simulink model "Latest_Greatest_vSandberg"  (R2022b)
settings: Solver=ode4  StartTime=0  StopTime=15  FixedStep=DeltaT  RelTol=1e-6  EnableMultiTasking=on
InitFcn:
  | %run('final_report_initexternal')
  | % Bifocal Relay Mirror Spacecraft (prior to payload installation) Dynamics Simulation          TA Sands
  | clear all;close all;clc;warning off all;
  | 
  | % Simulation run parameters
  | Rate=34.3; Rate=100;  DeltaT=1/Rate;
  | 
  | % Maneuver Parameters
  | roll=0;  pitch=0; yaw=30;   roll=roll*pi/180; pitch=pitch*pi/180; yaw=yaw*pi/180;
  | SlewStart=5; SlewTime=10; SACengage=0;
  | SlewStart=5; SlewTime=5;
  | t0=SlewTime;
  | tf=SlewTime+5;
  | %%
  | 
  | %Constants0
  | Re=6371.2e3;mu=398601.2e9;          %earth radius and universal gravitation constant
  | 
  | % tht=0.5*((sin(pi/SlewTime*(u(4)+2.5)))+1).*[u(1) u(2) u(3)]';
  | % w=(30/77.1239)*0.5*(pi/SlewTime)*((cos(pi/SlewTime*(u(4)+2.5)))+1).*[u(1) u(2) u(3)]'
  | % wdot=-(30/77.1239)*0.5*(pi/SlewTime)^(2)*((sin(pi/SlewTime*(u(4)+2.5)))).*[u(1) u(2) u(3)]'
  | 
  | %compare with differentiating in real time
  | 
  | % A0=[0 0 0];
  | % tht=A0+1/2*(1-cos(pi/SlewTime*(t-SlewStart)))*(A-A0);
  | % w=1/2*(pi/SlewTime)*sin(pi/SlewTime*(t-SlewStart))*(A-A0);
  | % wdot1=1/2*(pi/SlewTime)^2*cos(pi/SlewTime*(t-SlewStart))*(A-A0);
  | 
  | %Spacecraft orbit
  | h=0;                                     %orbit altitude
  | R=Re+h;                             %orbit radius from center of earth
  | we=0.000072921158553;   %earth's angular velocity rad/solar sec(Vallado)
  | wo=sqrt(mu/(Re+h)^3);        %orbit angular velocity
  | incln=36.6001*pi/180;          %Inclination assumed Monterey Latitude
  | epsilon=12*pi/180;  alphao=0;
  | uo=0; nuo=0;                        %Start S/C beneath subsolar point
  | betasun=60; gamma=1.5;
  | a=0.545491852; b=0.314939867;  c=0.704226952;   %Assumed spacecraft rectangular size
  | Area=[b*c a*c a*b];                 %projected area~m^2 in body x,y,z directions
  | density=4.39e-14;
  | kpre=-9.9639/24/3600/180*pi*0;      %nodal precession constant assumed zero here
  | wn=kpre*(Re/(Re+h))^3.5*cos(incln); %nodal precession (zero eccentricity)
  | V=wo*(Re+h);
  | rho=asin(Re/(h+Re));                %earth angular radius
  | Cd=2.5;     psun=4.5E-6;            %Drag coefficient and solar pressure constant~N/m^2
  | Kaero=-0.5*Cd*V^2;   Psolar=2*psun;  %constants for aero and solar torque calculation
  | dL=[0.002 0.002 0.008];             %predicted distance between cp and cg
  | Kme=2.3390e-005;
  | 
  | %Spacecraft Magnetic Properties (assumed)
  | mresid=[0 0 0.01];                  %Spacecraft residual magnetic moment
  | M=mresid;                           %Magnetic unit dipole vector
  | K=7.943e15;
  | 
  | %%
  | % Determining Principal Axes Frame
  | % ACTUAL Spacecraft Inertia conditions
  | Ix=16.67;   Iy=16.67;   Iz=16.67 ;
  | Ixy=0;  Iyz=0;  Ixz=0;
  | ... (+176 lines)
StopFcn:
  | toc
  | %run('final_report_stopexternal')
  | 
  | if flag==0; Hcmg=Hcmg;else;Hcmg=HcmgMP;end;
  | Hxcmg=[];Hycmg=[];Hzcmg=[];CondA=[]; CondA_MP=[];t=[]; SingPt=[];DetA=[];
  | for i=1:max(size(A));  t=[t i*DeltaT];  H=Hcmg(:,:,i); Hx=H(1,:);  Hy=H(2,:);  Hz=H(3,:);
  | detA=det(A(:,1:3,i));Hxcmg=[Hxcmg Hx];  Hycmg=[Hycmg Hy];  Hzcmg=[Hzcmg Hz];
  | CONDA=cond(A(:,:,i));
  | DetA=[DetA detA]; DetA=1./DetA;
  | CondA=[CondA CONDA];end;   %CondA=CondA./max(CondA); DetA=DetA./max(DetA);
  | Hmag=sqrt(Hxcmg.^2+Hycmg.^2+Hzcmg.^2);x=(max(t)-DeltaT);
  | 
  | InvCondA;
  | 
  | if flag==0; MaxInvCond=min(1./CondA(10*Rate+1:end));DELTA=delta;DELTAdot=deltadot;
  | else; MaxInvCond=min(1./CondA_MP(10*Rate+1:end));DELTA=delta_MP;DELTAdot=deltadot_MP;Hcmg=HcmgMP;end;
  | %
  | ERROR=(trajectory*180/pi-Euler);
  | 
  | figure(1); wdotTrajectory=[CMDTrajectory(:,1) CMDTrajectory(:,2) CMDTrajectory(:,3)];  wTrajectory=[CMDTrajectory(:,4) CMDTrajectory(:,5) CMDTrajectory(:,6)]; ThetaTrajectory=180/pi.*[trajectory(:,1) trajectory(:,2) trajectory(:,3)]; set(gca,'fontsize',32, 'fontname','Palatino Linotype');
  | subplot(3,1,1); plot(t,wdotTrajectory, 'linewidth',2); axis tight; grid; ylabel('\omega^d^o^t_C_M_D (deg)','fontsize',32); title('Desired Angle, Rate, Acceleration Trajectories','fontsize',32);   set(gca,'XTick',0:2:15);     set(gca,'XTickLabel',{' ',' ',' ',' ',' ',' ',' ',' ','15'}); set(gca,'fontsize',32, 'fontname','Palatino Linotype');
  | subplot(3,1,2); plot(t,wTrajectory,'linewidth',2); axis tight; grid; ylabel('\omega_C_M_D (deg)','fontsize',32);set(gca,'XTick',0:2:15);     set(gca,'XTickLabel',{' ',' ',' ',' ',' ',' ',' ',' ','15'}); set(gca,'fontsize',32, 'fontname','Palatino Linotype');
  | subplot(3,1,3); plot(t,ThetaTrajectory,'linewidth',2); axis tight; grid; ylabel('\theta_C_M_D (deg)','fontsize',32); xlabel('time (sec)','fontsize',32); set(gca,'fontsize',32, 'fontname','Palatino Linotype');
  | 
  | % figure(2);
  | % subplot(2,1,1);plot(t,Hmag,'LineWidth',3);   ylabel('|H_c_m_g|','Fontsize',16);grid;axis([0,x,0,3]); set(gca,'fontsize',16);set(gca,'XTickLabel',{' ',' ',' ',' ',' ',' ',' ',' ','15'});
  | % subplot(2,1,2);plot(t,InvCondA,'linewidth',3);grid;xlabel('t(sec)','fontsize',14,'fontname','times');ylabel('Cond[A]','fontsize',14,'fontname','times');axis([0,max(t),0,21.82]); set(gca,'fontsize',16);
  | %
  | % DELTA1=DELTA(1,:);DELTA2=DELTA(2,:);DELTA3=DELTA(3,:);DELTA4=DELTA(4,:);
  | % DELTAdot1=DELTAdot(1,:);DELTAdot2=DELTAdot(2,:);DELTAdot3=DELTAdot(3,:);DELTAdot4=DELTAdot(4,:);
  | %
  | % figure(3);subplot(4,1,1);plot(t,DELTA1,'LineWidth',3); title('Gimbal Angles','fontsize',16);ylabel('\theta_1(deg)','Fontsize',14);grid;axis tight; set(gca,'XTickLabel',{' ',' ',' ',' ',' ',' ',' ',' ','15'});set(gca,'fontsize',16);
  | % subplot(4,1,2);plot(t,DELTA2,'LineWidth',3); ylabel('\theta_2(deg)','Fontsize',16);grid;axis tight; set(gca,'XTickLabel',{' ',' ',' ',' ',' ',' ',' ',' ','15'});set(gca,'fontsize',16);
  | % subplot(4,1,3);plot(t,DELTA3,'LineWidth',3); ylabel('\theta_3(deg)','Fontsize',16);grid;axis tight; set(gca,'XTickLabel',{' ',' ',' ',' ',' ',' ',' ',' ','15'});set(gca,'fontsize',16);
  | % subplot(4,1,4);plot(t,InvCondA,'linewidth',3);grid;xlabel('t(sec)','fontsize',14,'fontname','times');ylabel('Cond[A]','fontsize',14,'fontname','times');axis([0,max(t),0,21.82]); set(gca,'fontsize',16);
  | %
  | % figure(4);subplot(4,1,1);plot(t,DELTAdot1,'LineWidth',3);  title('Gimbal Angle RATES','fontsize',16); ylabel('\theta_d_o_t_1(rad/s)','Fontsize',16);grid; axis([0,x,-pi*1.1,pi*1.1]);   set(gca,'XTickLabel',{' ',' ',' ',' ',' ',' ',' ',' ','15'});set(gca,'fontsize',16);
  | % subplot(4,1,2);plot(t,DELTAdot2,'LineWidth',3);   ylabel('\theta_d_o_t_2(rad/s)','Fontsize',16);grid;axis([0,x,-pi*1.1,pi*1.1]);   set(gca,'XTickLabel',{' ',' ',' ',' ',' ',' ',' ',' ','15'});   set(gca,'fontsize',16);
  | % subplot(4,1,3);plot(t,DELTAdot3,'LineWidth',3);   ylabel('\theta_d_o_t_3(rad/s)','Fontsize',16);grid;axis([0,x,-pi*1.1,pi*1.1]); set(gca,'XTickLabel',{' ',' ',' ',' ',' ',' ',' ',' ','15'});set(gca,'fontsize',16);
  | % subplot(4,1,4);plot(t,InvCondA,'linewidth',3);grid;xlabel('t(sec)','fontsize',14,'fontname','times');ylabel('Cond[A]','fontsize',14,'fontname','times');axis([0,max(t),0,21.82]); set(gca,'fontsize',16);
  | %
  | % figure(5);
  | % subplot(4,1,1);plot(t,Hxcmg,'linewidth',3);axis([0,x,-3.25,3.25]);grid;ylabel('h_x/|h|','fontsize',16);title('Normalized Momentum','fontsize',16);set(gca,'XTickLabel',{' ',' ',' ',' ',' ',' ',' ',' ','15'});set(gca,'fontsize',16);
  | % subplot(4,1,2);plot(t,Hycmg,'linewidth',3);axis([0,x,-3.25,3.25]);grid;ylabel('h_y/|h|','fontsize',16);set(gca,'XTickLabel',{' ',' ',' ',' ',' ',' ',' ',' ','15'});set(gca,'fontsize',16);
  | % subplot(4,1,3);plot(t,Hzcmg,'linewidth',3);axis([0,x,-3.25,3.25]);grid;ylabel('h_z/|h|','fontsize',16);  set(gca,'XTickLabel',{' ',' ',' ',' ',' ',' ',' ',' ','15'});set(gca,'fontsize',16);
  | % subplot(4,1,4);plot(t,InvCondA,'linewidth',3);grid;xlabel('t(sec)','fontsize',14,'fontname','times');ylabel('Cond[A]','fontsize',14,'fontname','times');axis([0,max(t),0,21.82]); set(gca,'fontsize',16);
  | %
  | figure(6); EulerX=Euler(:,1);EulerY=Euler(:,2);EulerZ=Euler(:,3);
  | subplot(4,1,1);plot(t,EulerX,'linewidth',3); axis([0,x,min(EulerX),max(EulerX)]);grid;ylabel('\phi(deg)','fontsize',32);title('True Euler Angles','fontsize',14);  set(gca,'XTickLabel',{' ',' ',' ',' ',' ',' ',' ',' ','15'});  set(gca,'fontsize',32, 'fontname','Palatino Linotype');
  | subplot(4,1,2);plot(t,EulerY,'linewidth',3);  axis([0,x,min(EulerY),max(EulerY)]); grid;ylabel('\theta(deg)','fontsize',32);  set(gca,'XTickLabel',{' ',' ',' ',' ',' ',' ',' ',' ','15'}); set(gca,'fontsize',32, 'fontname','Palatino Linotype');
  | subplot(4,1,3);plot(t,EulerZ,'linewidth',3);axis([0,x,min(EulerZ),max(EulerZ)]);grid;  ylabel('\psi(deg)','fontsize',32);  set(gca,'XTickLabel',{' ',' ',' ',' ',' ',' ',' ',' ','15'});  set(gca,'fontsize',32, 'fontname','Palatino Linotype');
  | subplot(4,1,4);plot(t,InvCondA,'linewidth',3);grid;xlabel('t(sec)','fontsize',32,'fontname','times');ylabel('Cond[A]','fontsize',14,'fontname','times');axis([0,max(t),0,21.82]); set(gca,'fontsize',32, 'fontname','Palatino Linotype');
  | 
  | EX=ERROR(:,1);  EY=ERROR(:,2);     EZ=ERROR(:,3);
  | MeanXerror=mean(EX); Xmean=num2str(MeanXerror); xmean=['\mu_\phi=', Xmean];
  | STDx=std(EX);Xsigma=num2str(STDx);SigmaX=['    \sigma_x=' Xsigma];  xlegend=[xmean, SigmaX];
  | MeanYerror=mean(EY); Ymean=num2str(MeanYerror); ymean=['\mu_\theta=', Ymean];
  | STDy=std(EY); Ysigma=num2str(STDy);SigmaY=['    \sigma_y=' Ysigma]; ylegend=[ymean, SigmaY];
  | MeanZerror=mean(EZ); Zmean=num2str(MeanZerror); zmean=['\mu_\psi=', Zmean];
  | STDz=std(EZ);Zsigma=num2str(STDz);SigmaZ=['    \sigma_z=' Zsigma]; zlegend=[zmean, SigmaZ];
  | ... (+113 lines)
undefined symbols (not defined in the file): magnitude, svd
libraries: vrlib x9, dspinverses x8, aerospace x5, matrix_library x4, simulink_need_slupdate x2, dspadpt3 x2
(part 3 of 4)

== system Latest_Greatest_vSandberg/Subsystem2/Subsystem/TAero & Tsolar ==
  note: Taero
  note: Tsolar
  note: Solar and Aero (Drag) Disturbances
  nu : Inport
  DCM : Inport  Port=2
  -1/2CdV^2 : Gain  Gain=-1/2*Cd*V^2  SaturateOnIntegerOverflow=on  OutDataTypeStr=Inherit: Same as input  ParamDataTypeStr=Inherit: Same as input
  2 3x1 cross product : aerospace/Axes Transformations/3x3 cross product
  2 3x1 cross product1 : aerospace/Axes Transformations/3x3 cross product
  Area : Constant  Value=[b*c,a*c,a*b]
  Atmospheric Density @ 800km : Constant  Value=density
  Atmospheric Force in Body Coords : Product  SaturateOnIntegerOverflow=on  OutDataTypeStr=Inherit: Same as first input
  Atmospheric Pressure in Body Coords : Product  SaturateOnIntegerOverflow=on  OutDataTypeStr=Inherit: Same as first input
  On/off : Gain  SaturateOnIntegerOverflow=on  OutDataTypeStr=Inherit: Same as input  ParamDataTypeStr=Inherit: Same as input
  On/off1 : Gain  SaturateOnIntegerOverflow=on  OutDataTypeStr=Inherit: Same as input  ParamDataTypeStr=Inherit: Same as input
  Product1 : Product  SaturateOnIntegerOverflow=on  OutDataTypeStr=Inherit: Same as first input
  Select ci1 : Subsystem
  Solar Force in body coordinates : Product  SaturateOnIntegerOverflow=on  OutDataTypeStr=Inherit: Same as first input
  Solar Pressure : Gain  Gain=Psolar  SaturateOnIntegerOverflow=on  OutDataTypeStr=Inherit: Same as input  ParamDataTypeStr=Inherit: Same as input
  Sum : Sum  SaturateOnIntegerOverflow=on
  Sun & Eclipse : Subsystem
  distance cp to cg : Constant  Value=-dL
  gamma^cos(nu)cos(B)-1 : Fcn  Expr=gamma^(cos(u[1])*cos(betasun)-1)
  Taero & Tsolar : Outport
  wires:
  gamma^cos(nu)cos(B)-1/1 -> Product1/1
  Atmospheric Density @ 800km/1 -> -1/2CdV^2/1
  -1/2CdV^2/1 -> Product1/2
  Solar Pressure/1 -> Solar Force in body coordinates/1
  Area/1 -> Solar Force in body coordinates/2, Atmospheric Force in Body Coords/1
  Product1/1 -> Atmospheric Pressure in Body Coords/1
  Select ci1/1(U(E)) -> Atmospheric Pressure in Body Coords/2
  Atmospheric Pressure in Body Coords/1 -> Atmospheric Force in Body Coords/2
  Solar Force in body coordinates/1 -> 2 3x1 cross product/1
  distance cp to cg/1 -> 2 3x1 cross product/2, 2 3x1 cross product1/2
  Sum/1 -> Taero & Tsolar/1
  Sun & Eclipse/1(Sb) -> Solar Pressure/1
  Sun & Eclipse/2(nu.) -> gamma^cos(nu)cos(B)-1/1
  DCM/1 -> Select ci1/1(U), Sun & Eclipse/2(DCM)
  On/off/1 -> Sum/2
  2 3x1 cross product1/1 -> On/off/1
  2 3x1 cross product/1 -> On/off1/1
  On/off1/1 -> Sum/1
  nu/1 -> Sun & Eclipse/1(nu)
  Atmospheric Force in Body Coords/1 -> 2 3x1 cross product1/1

== system Latest_Greatest_vSandberg/Subsystem2/Subsystem1/Gravity Gradient1 ==
  note: Cant forget that need to divide out by 3 to get the gravitational force
  note: Gravity Gradient Disturbances
  DCM : Inport
  r_body : Inport  Port=2
  3*mu/(norm(r)^3) : MATLABFcn  MATLABFcn=3*mu/norm(u)^3  OutputDimensions=1
  Body Inertia : Gain  Gain=Imo  Multiplication=Matrix(K*u)  SaturateOnIntegerOverflow=on  OutDataTypeStr=Inherit: Same as input  ParamDataTypeStr=Inherit: Same as input
  Cross Product : matrix_library/Cross Product
  Display : Display
  Gain : Gain  Gain=-m/3
  Product : Product
  Product1 : Product
  Select ci3 : Subsystem
  To Workspace2 : ToWorkspace  VariableName=r2  SampleTime=-1
  Tgg : Outport
  Fgg : Outport  Port=2
  wires:
  Gain/1 -> Display/1, Fgg/1
  DCM/1 -> To Workspace2/1, Select ci3/1(U)
  Select ci3/1(U(E)) -> Cross Product/1, Body Inertia/1
  Body Inertia/1 -> Cross Product/2
  Product/1 -> Tgg/1
  r_body/1 -> Product1/2, 3*mu/(norm(r)^3)/1
  Cross Product/1 -> Product/1
  3*mu/(norm(r)^3)/1 -> Product1/1, Product/2
  Product1/1 -> Gain/1

== system Latest_Greatest_vSandberg/Subsystem2/Subsystem1/Magnetic Torque ==
  note: Magnetic Disturbances
  note: Bzo
  note: Byo
  note: Bxo
  DCM : Inport
  alpha : Inport  Port=2
  inclination : Inport  Port=3
  u : Inport  Port=4
  .K/R^3 : Gain  Gain=K/R^3  SaturateOnIntegerOverflow=on  OutDataTypeStr=Inherit: Same as input  ParamDataTypeStr=Inherit: Same as input
  Cross Product : matrix_library/Cross Product
  Cx (orbit coordinates) : Fcn  Expr="cos(u[2])* ( cos(u[4])*sin(u[3])-sin(u[4])*cos(u[3])*cos(u[1])  ) - sin(u[2])*sin(u[4])*sin(u[1])"
  Cx (body coordinates) : Fcn  Expr=u[1]*u[10]+u[2]*u[11]+u[3]*u[12]
  Cy (orbit coordinates) : Fcn  Expr=-cos(u[4])*cos(u[3])-sin(u[4])*sin(u[3])*cos(u[1])
  Cy (body coordinates) : Fcn  Expr=u[4]*u[10]+u[5]*u[11]+u[6]*u[12]
  Cz (orbit coordinates) : Fcn  Expr="2*sin(u[2])*  (cos(u[4])*sin(u[3])-sin(u[4])*cos(u[3])*cos(u[1]) ) + 2*cos(u[2])*sin(u[4])*sin(u[1])"
  Cz (body coordinates) : Fcn  Expr=u[7]*u[10]+u[8]*u[11]+u[9]*u[12]
  Goto1 : Goto  TagVisibility=global
  K/R^3 : Gain  Gain=K/R^3  SaturateOnIntegerOverflow=on  OutDataTypeStr=Inherit: Same as input  ParamDataTypeStr=Inherit: Same as input
  K/R^3. : Gain  Gain=K/R^3  SaturateOnIntegerOverflow=on  OutDataTypeStr=Inherit: Same as input  ParamDataTypeStr=Inherit: Same as input
  Magnetic B Field : Scope  NumInputPorts=3
  Magnetic B Field in Body Coords : Scope
  Magnetic Residual : Constant  Value=M
  Mux : Mux
  Mux1 : Mux
  Mux2 : Mux  Inputs=3
  epsilon : Constant  Value=epsilon
  Sb : Outport
  wires:
  Mux2/1 -> Goto1/1, Magnetic B Field in Body Coords/1, Cross Product/2
  Magnetic Residual/1 -> Cross Product/1
  Cross Product/1 -> Sb/1
  Cz (body coordinates)/1 -> Mux2/3
  Cx (body coordinates)/1 -> Mux2/1
  Cy (body coordinates)/1 -> Mux2/2
  Mux1/1 -> Cz (body coordinates)/1, Cx (body coordinates)/1, Cy (body coordinates)/1
  .K/R^3/1 -> Magnetic B Field/3, Mux1/4
  K/R^3./1 -> Magnetic B Field/2, Mux1/3
  K/R^3/1 -> Magnetic B Field/1, Mux1/2
  DCM/1 -> Mux1/1
  Cz (orbit coordinates)/1 -> .K/R^3/1
  Cy (orbit coordinates)/1 -> K/R^3./1
  Cx (orbit coordinates)/1 -> K/R^3/1
  epsilon/1 -> Mux/4
  Mux/1 -> Cx (orbit coordinates)/1, Cy (orbit coordinates)/1, Cz (orbit coordinates)/1
  inclination/1 -> Mux/3
  alpha/1 -> Mux/2
  u/1 -> Mux/1

== system Latest_Greatest_vSandberg/Subsystem2/Subsystem1/Orbit parameters ==
  note: Orbit parameters
  note: nu=nuo-alpha
  note: alpha
  Clock : Clock
  Sum2 : Sum  Inputs=-+  InputSameDT=on  SaturateOnIntegerOverflow=on  OutDataTypeStr=Inherit: Same as first input
  Sum3 : Sum  InputSameDT=on  SaturateOnIntegerOverflow=on  OutDataTypeStr=Inherit: Same as first input
  Sum4 : Sum  InputSameDT=on  SaturateOnIntegerOverflow=on  OutDataTypeStr=Inherit: Same as first input
  alphao : Constant  Value=alphao
  inclination : Constant  Value=incln
  nuo : Constant  Value=nuo
  udot*t=t/365/360 : Gain  Gain=1/365.242/360  SaturateOnIntegerOverflow=on  OutDataTypeStr=Inherit: Same as input  ParamDataTypeStr=Inherit: Same as input
  uo : Constant  Value=uo
  wo : Gain  Gain=wo  SaturateOnIntegerOverflow=on  OutDataTypeStr=Inherit: Same as input  ParamDataTypeStr=Inherit: Same as input
  alpha : Outport
  incln : Outport  Port=2
  u : Outport  Port=3
  nu : Outport  Port=4
  wires:
  Sum3/1 -> u/1
  inclination/1 -> incln/1
  Sum2/1 -> nu/1
  Sum4/1 -> alpha/1, Sum2/2
  nuo/1 -> Sum2/1
  uo/1 -> Sum3/2
  udot*t=t/365/360/1 -> Sum3/1
  wo/1 -> Sum4/2
  alphao/1 -> Sum4/1
  Clock/1 -> udot*t=t/365/360/1, wo/1

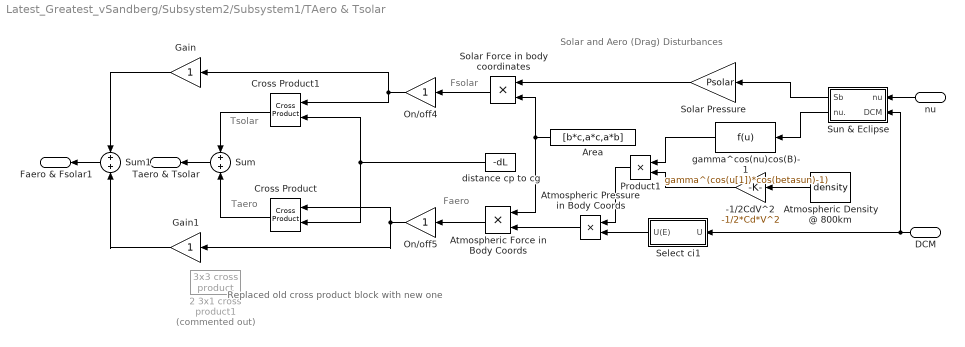
== system Latest_Greatest_vSandberg/Subsystem2/Subsystem1/TAero & Tsolar ==
  note: Fsolar
  note: Faero
  note: Solar and Aero (Drag) Disturbances
  note: Tsolar
  note: Taero
  note: Replaced old cross product block with new one
  nu : Inport
  DCM : Inport  Port=2
  -1/2CdV^2 : Gain  Gain=-1/2*Cd*V^2  SaturateOnIntegerOverflow=on  OutDataTypeStr=Inherit: Same as input  ParamDataTypeStr=Inherit: Same as input
  2 3x1 cross product1 : aerospace/Axes Transformations/3x3 cross product  Commented=on
  Area : Constant  Value=[b*c,a*c,a*b]
  Atmospheric Density @ 800km : Constant  Value=density
  Atmospheric Force in Body Coords : Product  SaturateOnIntegerOverflow=on  OutDataTypeStr=Inherit: Same as first input
  Atmospheric Pressure in Body Coords : Product  SaturateOnIntegerOverflow=on  OutDataTypeStr=Inherit: Same as first input
  Cross Product : vrlib/Utilities/Cross Product
  Cross Product1 : vrlib/Utilities/Cross Product
  Gain : Gain
  Gain1 : Gain
  On/off4 : Gain  SaturateOnIntegerOverflow=on  OutDataTypeStr=Inherit: Same as input  ParamDataTypeStr=Inherit: Same as input
  On/off5 : Gain  SaturateOnIntegerOverflow=on  OutDataTypeStr=Inherit: Same as input  ParamDataTypeStr=Inherit: Same as input
  Product1 : Product  SaturateOnIntegerOverflow=on  OutDataTypeStr=Inherit: Same as first input
  Select ci1 : Subsystem
  Solar Force in body coordinates : Product  SaturateOnIntegerOverflow=on  OutDataTypeStr=Inherit: Same as first input
  Solar Pressure : Gain  Gain=Psolar  SaturateOnIntegerOverflow=on  OutDataTypeStr=Inherit: Same as input  ParamDataTypeStr=Inherit: Same as input
  Sum : Sum  SaturateOnIntegerOverflow=on
  Sum1 : Sum  SaturateOnIntegerOverflow=on
  Sun & Eclipse : Subsystem
  distance cp to cg : Constant  Value=-dL
  gamma^cos(nu)cos(B)-1 : Fcn  Expr=gamma^(cos(u[1])*cos(betasun)-1)
  Taero & Tsolar : Outport
  Faero & Fsolar1 : Outport  Port=2
  wires:
  Gain1/1 -> Sum1/2
  Gain/1 -> Sum1/1
  On/off4/1 -> Gain/1, Cross Product1/1
  On/off5/1 -> Gain1/1, Cross Product/1
  Atmospheric Force in Body Coords/1 -> On/off5/1
  Solar Force in body coordinates/1 -> On/off4/1
  Sum1/1 -> Faero & Fsolar1/1
  nu/1 -> Sun & Eclipse/1(nu)
  Cross Product1/1 -> Sum/1
  Cross Product/1 -> Sum/2
  DCM/1 -> Sun & Eclipse/2(DCM), Select ci1/1(U)
  Sun & Eclipse/2(nu.) -> gamma^cos(nu)cos(B)-1/1
  Sun & Eclipse/1(Sb) -> Solar Pressure/1
  Sum/1 -> Taero & Tsolar/1
  distance cp to cg/1 -> Cross Product/2, Cross Product1/2
  Atmospheric Pressure in Body Coords/1 -> Atmospheric Force in Body Coords/2
  Select ci1/1(U(E)) -> Atmospheric Pressure in Body Coords/2
  Product1/1 -> Atmospheric Pressure in Body Coords/1
  Area/1 -> Solar Force in body coordinates/2, Atmospheric Force in Body Coords/1
  Solar Pressure/1 -> Solar Force in body coordinates/1
  -1/2CdV^2/1 -> Product1/2
  Atmospheric Density @ 800km/1 -> -1/2CdV^2/1
  gamma^cos(nu)cos(B)-1/1 -> Product1/1

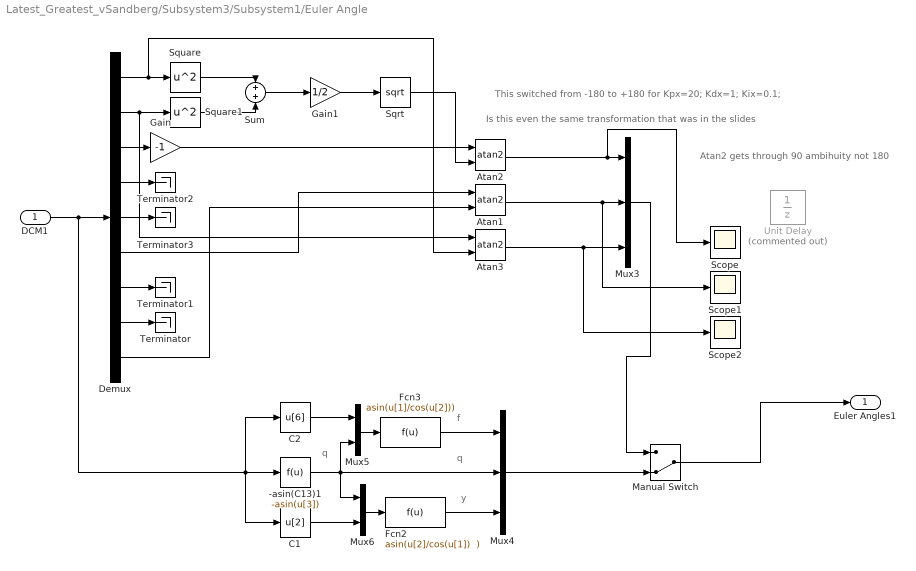
== system Latest_Greatest_vSandberg/Subsystem3/Subsystem1/Euler Angle ==
  note: Atan2 gets through 90 ambihuity not 180
  note: Is this even the same transformation that was in the slides
  note: f
  note: This switched from -180 to +180 for Kpx=20; Kdx=1; Kix=0.1;
  note: q
  note: q
  note: y
  DCM1 : Inport
  -asin(C13)1 : Fcn  Expr=-asin(u[3])
  Atan1 : Trigonometry  Operator=atan2
  Atan2 : Trigonometry  Operator=atan2
  Atan3 : Trigonometry  Operator=atan2
  C1 : Fcn  Expr=u[2]
  C2 : Fcn  Expr=u[6]
  Demux : Demux  Outputs=9
  Fcn2 : Fcn  Expr="asin(u[2]/cos(u[1])  )"
  Fcn3 : Fcn  Expr=asin(u[1]/cos(u[2]))
  Gain : Gain  Gain=-1
  Gain1 : Gain  Gain=1/2
  Manual Switch : ManualSwitch  CurrentSetting=0
  Mux3 : Mux  Inputs=3
  Mux4 : Mux  Inputs=3
  Mux5 : Mux  Inputs=2
  Mux6 : Mux  Inputs=2
  Scope : Scope
  Scope1 : Scope
  Scope2 : Scope
  Sqrt : Sqrt
  Square : Math  Operator=square
  Square1 : Math  Operator=square
  Sum : Sum
  Terminator{,1..3} (4 alike) : Terminator
  Unit Delay : UnitDelay  Commented=on  SampleTime=-1  HasFrameUpgradeWarning=on
  Euler Angles1 : Outport  VectorParamsAs1DForOutWhenUnconnected=off
  wires:
  DCM1/1 -> -asin(C13)1/1, C2/1, C1/1, Demux/1
  Square1/1 -> Sum/2
  -asin(C13)1/1 -> Mux4/2, Mux5/2, Mux6/1
  Gain1/1 -> Sqrt/1
  C2/1 -> Mux5/1
  Fcn3/1 -> Mux4/1
  Demux/3 -> Gain/1
  Mux5/1 -> Fcn3/1
  Mux3/1 -> Manual Switch/1
  Gain/1 -> Atan2/1
  Demux/6 -> Atan1/1
  Mux4/1 -> Manual Switch/2
  Demux/7 -> Terminator1/1
  Sqrt/1 -> Atan2/2
  Demux/9 -> Atan1/2
  C1/1 -> Mux6/2
  Demux/8 -> Terminator/1
  Atan1/1 -> Scope1/1, Mux3/2
  Demux/1 -> Atan3/2, Square/1
  Demux/2 -> Atan3/1, Square1/1
  Square/1 -> Sum/1
  Sum/1 -> Gain1/1
  Fcn2/1 -> Mux4/3
  Demux/5 -> Terminator3/1
  Manual Switch/1 -> Euler Angles1/1
  Demux/4 -> Terminator2/1
  Atan3/1 -> Scope2/1, Mux3/3
  Mux6/1 -> Fcn2/1
  Atan2/1 -> Scope/1, Mux3/1

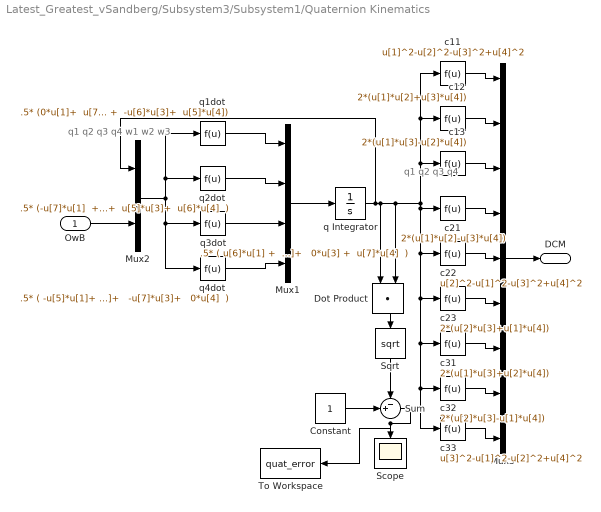
== system Latest_Greatest_vSandberg/Subsystem3/Subsystem1/Quaternion Kinematics ==
  note: q1
      | q2
      | q3
      | q4
      | w1
      | w2
      | w3
  note: q1
      | q2
      | q3
      | q4
  OwB : Inport
  Constant : Constant
  Dot Product : DotProduct  OutDataTypeStr=Inherit: Inherit via internal rule
  Mux1 : Mux
  Mux2 : Mux  Inputs=2
  Mux3 : Mux  Inputs=9
  Scope : Scope
  Sqrt : Sqrt
  Sum : Sum  Inputs=-+|
  To Workspace : ToWorkspace  VariableName=quat_error  SampleTime=-1
  c11 : Fcn  Expr=u[1]^2-u[2]^2-u[3]^2+u[4]^2
  c12 : Fcn  Expr=2*(u[1]*u[2]+u[3]*u[4])
  c13 : Fcn  Expr=2*(u[1]*u[3]-u[2]*u[4])
  c21 : Fcn  Expr=2*(u[1]*u[2]-u[3]*u[4])
  c22 : Fcn  Expr=u[2]^2-u[1]^2-u[3]^2+u[4]^2
  c23 : Fcn  Expr=2*(u[2]*u[3]+u[1]*u[4])
  c31 : Fcn  Expr=2*(u[1]*u[3]+u[2]*u[4])
  c32 : Fcn  Expr=2*(u[2]*u[3]-u[1]*u[4])
  c33 : Fcn  Expr=u[3]^2-u[1]^2-u[2]^2+u[4]^2
  q Integrator : Integrator  InitialCondition=qo
  q1dot : Fcn  Expr=".5* (0*u[1]+  u[7]*u[2] +  -u[6]*u[3]+  u[5]*u[4])"
  q2dot : Fcn  Expr=".5* (-u[7]*u[1]  +  0*u[2]+  u[5]*u[3]+  u[6]*u[4]  )"
  q3dot : Fcn  Expr=".5* ( u[6]*u[1] +  -u[5]*u[2]+   0*u[3] +  u[7]*u[4]  )"
  q4dot : Fcn  Expr=".5* ( -u[5]*u[1]+   -u[6]*u[2]+   -u[7]*u[3]+   0*u[4]  )"
  DCM : Outport  VectorParamsAs1DForOutWhenUnconnected=off
  wires:
  OwB/1 -> Mux2/2
  q1dot/1 -> Mux1/1
  q2dot/1 -> Mux1/2
  q3dot/1 -> Mux1/3
  q4dot/1 -> Mux1/4
  Mux1/1 -> q Integrator/1
  q Integrator/1 -> Dot Product/1, Dot Product/2, c12/1, c11/1, c13/1, c21/1, c22/1, c23/1, c31/1, c33/1, c32/1, Mux2/1
  c11/1 -> Mux3/1
  c12/1 -> Mux3/2
  c13/1 -> Mux3/3
  c22/1 -> Mux3/5
  c21/1 -> Mux3/4
  c23/1 -> Mux3/6
  c31/1 -> Mux3/7
  c32/1 -> Mux3/8
  c33/1 -> Mux3/9
  Mux3/1 -> DCM/1
  Mux2/1 -> q2dot/1, q1dot/1, q3dot/1, q4dot/1
  Dot Product/1 -> Sqrt/1
  Sqrt/1 -> Sum/1
  Sum/1 -> To Workspace/1, Scope/1
  Constant/1 -> Sum/2

== system Latest_Greatest_vSandberg/Subsystem3/Subsystem1/Select ci2 ==
  U : Inport
  C12 : Fcn  Expr=u[2]
  C22 : Fcn  Expr=u[5]
  C32 : Fcn  Expr=u[8]
  Mux2 : Mux  Inputs=3
  U(E) : Outport  VectorParamsAs1DForOutWhenUnconnected=off
  wires:
  C12/1 -> Mux2/1
  C22/1 -> Mux2/2
  C32/1 -> Mux2/3
  U/1 -> C32/1, C22/1, C12/1
  Mux2/1 -> U(E)/1

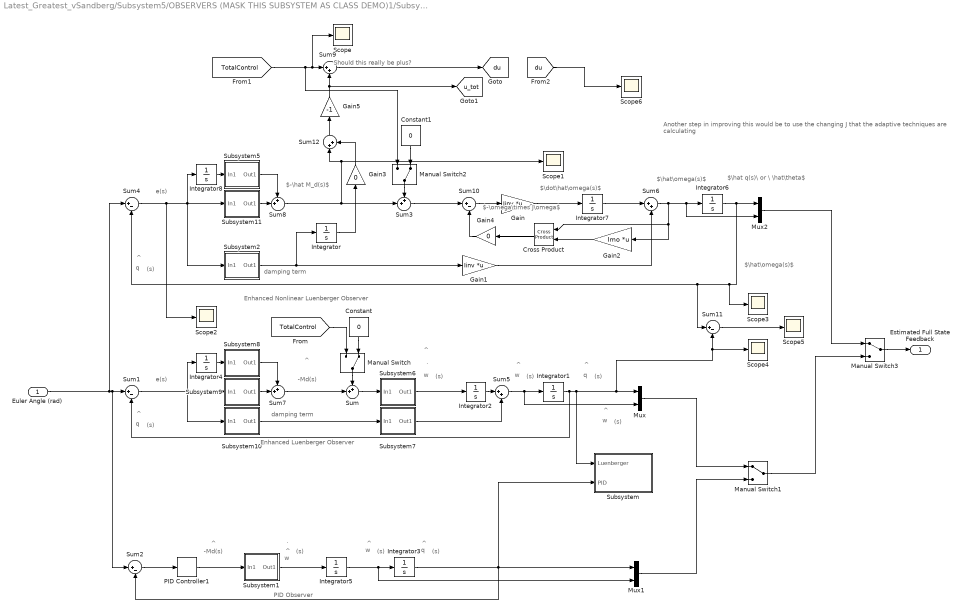
== system Latest_Greatest_vSandberg/Subsystem5/OBSERVERS (MASK THIS SUBSYSTEM AS CLASS DEMO)1/Subsystem ==
  note: Another step in improving this would be to use the changing J that the adaptive techniques are calculating
  note: Should this really be plus?
  note: PID Observer
  note: -Md(s)
  note: ^
  note: ^
  note: (s)
  note: w
  note: (s)
  note: .
  note: ^
  note: w
  note: e(s)
  note: q
  note: ^
  note: (s)
  note: ^
  note: (s)
  note: w
  note: damping term
  note: Enhanced Luenberger Observer
  note: ^
  note: (s)
  note: w
  note: (s)
  note: .
  note: ^
  note: w
  note: (s)
  note: ^
  note: q
  note: ^
  note: -Md(s)
  note: (s)
  note: ^
  note: q
  note: Enhanced Nonlinear Luenberger Observer
  note: $\hat q(s)\ or \ \hat\theta$
  note: q
  note: e(s)
  note: $-\hat M_d(s)$
  note: $\dot\hat\omega(s)$
  note: $\hat\omega(s)$
  note: damping term
  note: (s)
  note: ^
  note: $\hat\omega(s)$
  note: $-\omega\times J\omega$
  Euler Angle (rad) : Inport
  Constant : Constant  Value=0
  Constant1 : Constant  Value=0
  Cross Product : vrlib/Utilities/Cross Product
  Gain : Gain  Gain=Iinv  Multiplication=Matrix(K*u)
  Gain1 : Gain  Gain=Iinv  Multiplication=Matrix(K*u)
  Gain2 : Gain  Gain=Imo  Multiplication=Matrix(K*u)
  Gain3 : Gain  Gain=0
  Gain4 : Gain  Gain=0
  Gain5 : Gain  Gain=-1
  Integrator{,1..8} (9 alike) : Integrator
  Manual Switch : ManualSwitch  CurrentSetting=0
  Manual Switch1 : ManualSwitch
  Manual Switch2 : ManualSwitch  CurrentSetting=0
  Manual Switch3 : ManualSwitch
  Mux : Mux  Inputs=2
  Mux1 : Mux  Inputs=2
  Mux2 : Mux  Inputs=2
  PID Controller1 : simulink_need_slupdate/PID Controller  P=Kpo  I=Kio  D=Kdo
  Scope{,1..6} (7 alike) : Scope
  Subsystem : Subsystem
      mask Display: disp('Scopes')
  Subsystem1 : Subsystem
      mask Display: disp('1/J^p')
  Subsystem10 : Subsystem
      mask Display: disp('Kdo')
  Subsystem11 : Subsystem
      mask Display: disp('Kpo')
  Subsystem2 : Subsystem
      mask Display: disp('Kdo')
  Subsystem5 : Subsystem
      mask Display: disp('Kio')
  Subsystem6 : Subsystem
      mask Display: disp('1/J^p')
  Subsystem7 : Subsystem
      mask Display: disp('1/J^p')
  Subsystem8 : Subsystem
      mask Display: disp('Kio')
  Subsystem9 : Subsystem
      mask Display: disp('Kpo')
  Sum{,3,7..8} (4 alike) : Sum  Inputs=++|
  Sum{1..2,4,10..11} (5 alike) : Sum  Inputs=|+-
  Sum{5..6,9,12} (4 alike) : Sum  Inputs=|++
  Estimated Full State Feedback : Outport  VectorParamsAs1DForOutWhenUnconnected=off
  tag scope: du=global, u_tot=global
  wires:
  Mux1/1 -> Manual Switch1/2
  Mux/1 -> Manual Switch1/1
  PID Controller1/1 -> Subsystem1/1(In1)
  Integrator3/1 -> Mux1/1, Subsystem/2(PID), Sum2/2
  Integrator5/1 -> Mux1/2, Integrator3/1
  Subsystem1/1(Out1) -> Integrator5/1
  Manual Switch/1 -> Sum/1
  Constant/1 -> Manual Switch/2
  [TotalControl] -> Manual Switch/1
  Sum1/1 -> Subsystem10/1(In1), Subsystem9/1(In1), Integrator4/1
  Sum/1 -> Subsystem6/1(In1)
  Sum7/1 -> Sum/2
  Integrator1/1 -> Subsystem/1(Luenberger), Scope4/1, Sum11/2, Mux/1, Sum1/2
  Sum5/1 -> Mux/2, Integrator1/1
  Integrator4/1 -> Subsystem8/1(In1)
  Subsystem10/1(Out1) -> Subsystem7/1(In1)
  Subsystem9/1(Out1) -> Sum7/2
  Subsystem8/1(Out1) -> Sum7/1
  Subsystem7/1(Out1) -> Sum5/2
  Integrator2/1 -> Sum5/1
  Subsystem6/1(Out1) -> Integrator2/1
  Sum2/1 -> PID Controller1/1
  Manual Switch3/1 -> Estimated Full State Feedback/1
  Mux2/1 -> Manual Switch3/1
  Integrator8/1 -> Subsystem5/1(In1)
  [TotalControl] -> Manual Switch2/1, Scope/1, Sum9/1
  Sum8/1 -> Sum12/1, Scope1/1, Sum3/2
  Constant1/1 -> Manual Switch2/2
  Gain1/1 -> Sum6/2
  Subsystem11/1(Out1) -> Sum8/2
  Integrator6/1 -> Mux2/1, Scope3/1, Sum11/1, Sum4/2
  Subsystem2/1(Out1) -> Integrator/1, Gain1/1
  Sum6/1 -> Gain2/1, Cross Product/1, Mux2/2, Integrator6/1
  Euler Angle (rad)/1 -> Sum1/1, Sum2/1, Sum4/1
  Sum4/1 -> Scope2/1, Subsystem2/1(In1), Subsystem11/1(In1), Integrator8/1
  Integrator7/1 -> Sum6/1
  Subsystem5/1(Out1) -> Sum8/1
  Gain/1 -> Integrator7/1
  Manual Switch2/1 -> Sum3/1
  Gain2/1 -> Cross Product/2
  Cross Product/1 -> Gain4/1
  Sum10/1 -> Gain/1
  Sum3/1 -> Sum10/1
  Sum11/1 -> Scope5/1
  [du] -> Scope6/1
  Integrator/1 -> Gain3/1
  Sum9/1 -> [du]
  Gain3/1 -> Sum12/2
  Gain4/1 -> Sum10/2
  Manual Switch1/1 -> Manual Switch3/2
  Sum12/1 -> Gain5/1
  Gain5/1 -> [u_tot], Sum9/2

== system Latest_Greatest_vSandberg/CMGs/Subsystem3/Subsystem1/Subsystem25 ==
  In1 : Inport
  Clock : Clock
  Ki : Gain  Gain=-Ki
  To Workspace : ToWorkspace  VariableName=t  SampleTime=-1
  Out1 : Outport  VectorParamsAs1DForOutWhenUnconnected=off
  wires:
  Clock/1 -> To Workspace/1
  In1/1 -> Ki/1
  Ki/1 -> Out1/1

== system Latest_Greatest_vSandberg/CMGs/Subsystem3/Subsystem1/Subsystem26 ==
  In1 : Inport
  Gain : Gain  Gain=-Kp
  Out1 : Outport  VectorParamsAs1DForOutWhenUnconnected=off
  wires:
  Gain/1 -> Out1/1
  In1/1 -> Gain/1

== system Latest_Greatest_vSandberg/CMGs/Subsystem3/Subsystem1/Subsystem27 ==
  In1 : Inport
  Gain : Gain  Gain=-Kd
  Out1 : Outport  VectorParamsAs1DForOutWhenUnconnected=off
  wires:
  In1/1 -> Gain/1
  Gain/1 -> Out1/1

== system Latest_Greatest_vSandberg/CMGs/Subsystem3/Subsystem4/Subsystem ==
  note: I*wdot+wxI*w
  In1 : Inport
  In2 : Inport  Port=2
  Cross Product : vrlib/Utilities/Cross Product
  Gain : Gain  Gain=Imo  Multiplication=Matrix(K*u)
  Gain1 : Gain  Gain=Imo  Multiplication=Matrix(K*u)
  Sum : Sum  Inputs=|++
  Out1 : Outport
  wires:
  In1/1 -> Gain/1
  Gain1/1 -> Cross Product/2
  Gain/1 -> Sum/1
  Sum/1 -> Out1/1
  In2/1 -> Gain1/1, Cross Product/1
  Cross Product/1 -> Sum/2

== system Latest_Greatest_vSandberg/CMGs/Subsystem3/Subsystem4/Subsystem1 ==
  note: REMAKE THIS< WITH AND WITHOUT REFERENCE
  note: xdotr
  note: xdDot
  note: F
  note: -G
  note: F
  note: s
  note: =
  note: .
  note: ^
  note: q
  omegadot_traj : Inport
  w : Inport  Port=2
  LAMBDA*xtilda : Inport  Port=3
  -G : Gain  Gain=-ETA  SaturateOnIntegerOverflow=on  OutDataTypeStr=Inherit: Same as input  ParamDataTypeStr=Inherit: Same as input
  Derivative2 : Derivative
  F : MATLABFcn  MATLABFcn="[u(1) u(2) u(3) 0 0 0 0 -u(6) u(5);  0 u(1) 0 u(2) u(3) 0 u(6) 0 u(4);  0 0 u(1) 0 u(2) u(3) -u(5) u(4) 0  ]"  OutputDimensions=[27]
  Integrator11 : Integrator  InitialCondition=THETAo
  Manual Switch3 : ManualSwitch
  Math Function : Math  Operator=transpose  SignedPower=on
  Mux : Mux  Inputs=2
  Reshape : Reshape  OutputDimensionality=Customize  OutputDimensions=[3,9]
  Reshape1 : Reshape  OutputDimensions=[1,9]
  Scope{,1..3} (4 alike) : Scope
  Sum2 : Sum  Inputs=|-+  SaturateOnIntegerOverflow=on
  To Workspace : ToWorkspace  VariableName=THETAhat  SampleTime=-1
  To Workspace1 : ToWorkspace  VariableName=CMDTrajectory  SampleTime=-1
  "[F] {q}" : Product  Multiplication=Matrix(*)
  "[PHI] {s}" : Product  Multiplication=Matrix(*)  SaturateOnIntegerOverflow=on  OutDataTypeStr=Inherit: Same as first input
  l : Gain  Gain=LAMBDA  SaturateOnIntegerOverflow=on  OutDataTypeStr=Inherit: Same as input  ParamDataTypeStr=Inherit: Same as input
  l2 : Gain  Gain=uffGain  SaturateOnIntegerOverflow=on  OutDataTypeStr=Inherit: Same as input  ParamDataTypeStr=Inherit: Same as input
  rad2deg : Gain  Gain=180/pi  SaturateOnIntegerOverflow=on  OutDataTypeStr=Inherit: Same as input  ParamDataTypeStr=Inherit: Same as input
  Out1 : Outport
  wires:
  omegadot_traj/1 -> Manual Switch3/1
  Derivative2/1 -> Manual Switch3/2
  Math Function/1 -> "[PHI] {s}"/1
  l/1 -> Sum2/1
  "[PHI] {s}"/1 -> -G/1
  -G/1 -> Integrator11/1
  Reshape1/1 -> To Workspace/1
  Manual Switch3/1 -> Mux/1, Scope1/1
  Sum2/1 -> Scope3/1, "[PHI] {s}"/2
  F/1 -> Reshape/1
  l2/1 -> Out1/1
  Integrator11/1 -> Scope2/1, "[F] {q}"/2, Reshape1/1
  Reshape/1 -> "[F] {q}"/1, Math Function/1
  w/1 -> Sum2/2, Mux/2, Derivative2/1
  rad2deg/1 -> To Workspace1/1
  Mux/1 -> F/1, rad2deg/1
  "[F] {q}"/1 -> Scope/1, l2/1
  LAMBDA*xtilda/1 -> l/1

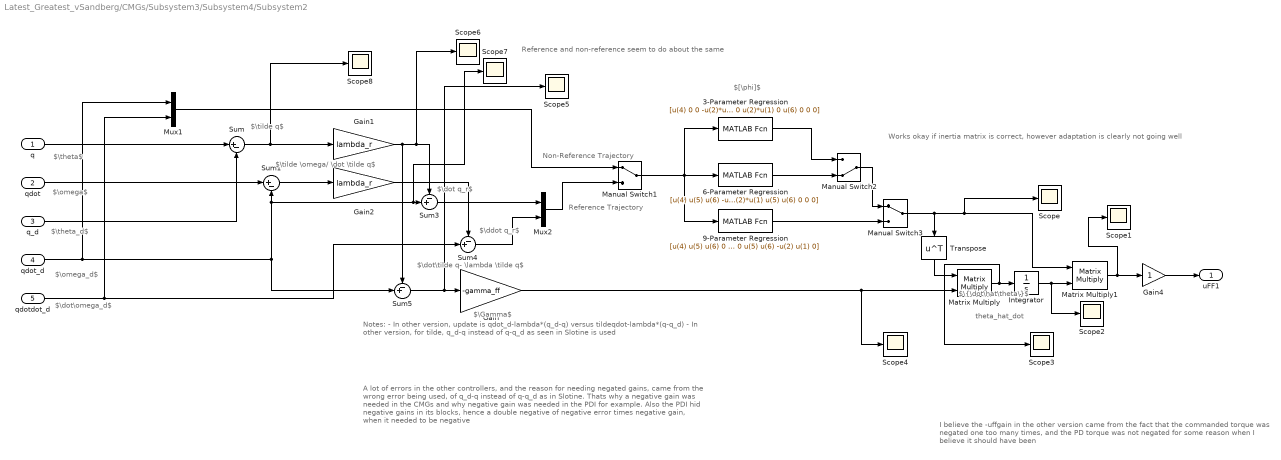
== system Latest_Greatest_vSandberg/CMGs/Subsystem3/Subsystem4/Subsystem2 ==
  note: Reference and non-reference seem to do about the same
  note: A lot of errors in the other controllers, and the reason for needing negated gains, came from the wrong error being used, of q_d-q instead of q-q_d as in Slotine. Thats why a negative gain was needed in the CMGs and why negative gain was needed in the PDI for example. Also the PDI hid negative gains in its blocks, hence a double negative of negative error times negative gain, when it needed to be negative
  note: I believe the -uffgain in the other version came from the fact that the commanded torque was negated one too many times, and the PD torque was not negated for some reason when I believe it should have been
  note: Notes:
      | - In other version, update is qdot_d-lambda*(q_d-q) versus tildeqdot-lambda*(q-q_d)
      | - In other version, for tilde, q_d-q instead of q-q_d as seen in Slotine is used
  note: Works okay if inertia matrix is correct, however adaptation is clearly not going well
  note: theta_hat_dot
  note: $\{\dot\hat\theta\}$
  note: $\Gamma$
  note: $\dot\tilde q- \lambda \tilde q$
  note: $[\phi]$
  note: Non-Reference Trajectory
  note: Reference Trajectory
  note: $\dot q_r$
  note: $\ddot q_r$
  note: $\tilde \omega/ \dot \tilde q$
  note: $\theta$
  note: $\omega$
  note: $\theta_d$
  note: $\omega_d$
  note: $\dot\omega_d$
  note: $\tilde q$
  q : Inport
  qdot : Inport  Port=2
  q_d : Inport  Port=3
  qdot_d : Inport  Port=4
  qdotdot_d : Inport  Port=5
  3-Parameter Regression : MATLABFcn  MATLABFcn=[u(4) 0 0 -u(2)*u(3) 0 u(3)*u(2) 0 0 0;u(1)*u(3) 0 0 u(5) 0 -u(3)*u(1) 0 0 0;-u(1)*u(2) 0 0 u(2)*u(1) 0 u(6) 0 0 0]  Output1D=off
  6-Parameter Regression : MATLABFcn  MATLABFcn=[u(4) u(5) u(6) -u(2)*u(3) 0 u(3)*u(2) 0 0 0;u(1)*u(3) u(4) 0 u(5) u(6) -u(3)*u(1) 0 0 0;-u(1)*u(2) 0 u(4) u(2)*u(1) u(5) u(6) 0 0 0]  Output1D=off
  9-Parameter Regression : MATLABFcn  MATLABFcn=[u(4) u(5) u(6) 0 0 0 0 -u(3) u(2);0 u(4) 0 u(5) u(6) 0 u(3) 0 u(1);0 0 u(4) 0 u(5) u(6) -u(2) u(1) 0]  Output1D=off
  Gain : Gain  Gain=-gamma_ff
  Gain1 : Gain  Gain=lambda_r
  Gain2 : Gain  Gain=lambda_r
  Gain4 : Gain
  Integrator : Integrator  InitialCondition=theta0'
  Manual Switch1 : ManualSwitch
  Manual Switch2 : ManualSwitch  CurrentSetting=0
  Manual Switch3 : ManualSwitch
  Matrix Multiply : Product  Multiplication=Matrix(*)
  Matrix Multiply1 : Product  Multiplication=Matrix(*)
  Mux1 : Mux  Inputs=2
  Mux2 : Mux  Inputs=2
  Scope{,1..8} (9 alike) : Scope
  Sum : Sum  Inputs=|+-
  Sum1 : Sum  Inputs=|+-
  Sum3 : Sum  Inputs=-+|
  Sum4 : Sum  Inputs=-+|
  Sum5 : Sum  Inputs=-+|
  Transpose : Math  Operator=transpose
  uFF1 : Outport  VectorParamsAs1DForOutWhenUnconnected=off
  wires:
  6-Parameter Regression/1 -> Manual Switch2/2
  9-Parameter Regression/1 -> Manual Switch3/2
  Sum/1 -> Scope8/1, Gain1/1
  Manual Switch3/1 -> Scope/1, Matrix Multiply1/1, Transpose/1
  Mux2/1 -> Manual Switch1/2
  Matrix Multiply1/1 -> Scope1/1, Gain4/1
  Manual Switch1/1 -> 3-Parameter Regression/1, 9-Parameter Regression/1, 6-Parameter Regression/1
  3-Parameter Regression/1 -> Manual Switch2/1
  q_d/1 -> Sum/2
  Transpose/1 -> Matrix Multiply/1
  q/1 -> Sum/1
  Gain/1 -> Scope4/1, Matrix Multiply/2
  Matrix Multiply/1 -> Scope3/1, Integrator/1
  Manual Switch2/1 -> Manual Switch3/1
  Mux1/1 -> Manual Switch1/1
  Integrator/1 -> Scope2/1, Matrix Multiply1/2
  Sum1/1 -> Gain2/1
  Sum3/1 -> Mux2/1
  qdot/1 -> Sum1/1
  Gain2/1 -> Sum4/1
  Sum4/1 -> Mux2/2
  Gain4/1 -> uFF1/1
  qdot_d/1 -> Sum5/2, Sum1/2, Scope7/1, Sum3/2, Mux1/1
  qdotdot_d/1 -> Mux1/2, Sum4/2
  Sum5/1 -> Scope5/1, Gain/1
  Gain1/1 -> Sum5/1, Scope6/1, Sum3/1

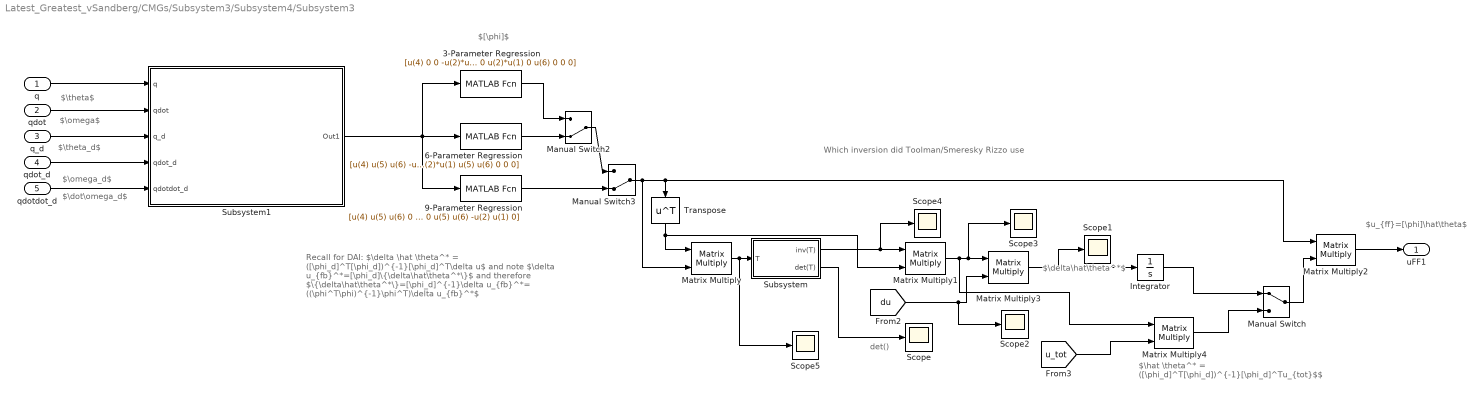
== system Latest_Greatest_vSandberg/CMGs/Subsystem3/Subsystem4/Subsystem3 ==
  note: $\hat \theta^* = ([\phi_d]^T[\phi_d])^{-1}[\phi_d]^Tu_{tot}$$
  note: Which inversion did Toolman/Smeresky Rizzo use
  note: $u_{ff}=[\phi]\hat\theta$
  note: $\delta\hat\theta^*$
  note: det()
  note: Recall for DAI:
      | $\delta \hat \theta^* = ([\phi_d]^T[\phi_d])^{-1}[\phi_d]^T\delta u$
      |
      | and note
      | $\delta u_{fb}^*=[\phi_d]\{\delta\hat\theta^*\}$ and therefore
      | $\{\delta\hat\theta^*\}=[\phi_d]^{-1}\delta u_{fb}^*= ((\phi^T\phi)^{-1}\phi^T)\delta u_{fb}^*$
  note: $\dot\omega_d$
  note: $\omega_d$
  note: $\theta_d$
  note: $\omega$
  note: $\theta$
  note: $[\phi]$
  q : Inport
  qdot : Inport  Port=2
  q_d : Inport  Port=3
  qdot_d : Inport  Port=4
  qdotdot_d : Inport  Port=5
  3-Parameter Regression : MATLABFcn  MATLABFcn=[u(4) 0 0 -u(2)*u(3) 0 u(3)*u(2) 0 0 0;u(1)*u(3) 0 0 u(5) 0 -u(3)*u(1) 0 0 0;-u(1)*u(2) 0 0 u(2)*u(1) 0 u(6) 0 0 0]  Output1D=off
  6-Parameter Regression : MATLABFcn  MATLABFcn=[u(4) u(5) u(6) -u(2)*u(3) 0 u(3)*u(2) 0 0 0;u(1)*u(3) u(4) 0 u(5) u(6) -u(3)*u(1) 0 0 0;-u(1)*u(2) 0 u(4) u(2)*u(1) u(5) u(6) 0 0 0]  Output1D=off
  9-Parameter Regression : MATLABFcn  MATLABFcn=[u(4) u(5) u(6) 0 0 0 0 -u(3) u(2);0 u(4) 0 u(5) u(6) 0 u(3) 0 u(1);0 0 u(4) 0 u(5) u(6) -u(2) u(1) 0]  Output1D=off
  Integrator : Integrator  InitialCondition=theta0
  Manual Switch : ManualSwitch
  Manual Switch2 : ManualSwitch  CurrentSetting=0
  Manual Switch3 : ManualSwitch  CurrentSetting=0
  Matrix Multiply{,1..4} (5 alike) : Product  Multiplication=Matrix(*)
  Scope{,1..5} (6 alike) : Scope
  Subsystem : Subsystem
      mask Display: disp('Invert Matrix')
  Subsystem1 : Subsystem
      mask Display: disp('Full State')
  Transpose : Math  Operator=transpose
  uFF1 : Outport  VectorParamsAs1DForOutWhenUnconnected=off
  wires:
  Transpose/1 -> Matrix Multiply/1, Matrix Multiply1/2
  Manual Switch2/1 -> Manual Switch3/1
  Matrix Multiply/1 -> Scope5/1, Subsystem/1(T)
  3-Parameter Regression/1 -> Manual Switch2/1
  Manual Switch3/1 -> Matrix Multiply/2, Matrix Multiply2/1, Transpose/1
  9-Parameter Regression/1 -> Manual Switch3/2
  6-Parameter Regression/1 -> Manual Switch2/2
  Subsystem/1(inv(T)) -> Scope4/1, Matrix Multiply1/1
  Subsystem/2(det(T)) -> Scope/1
  Subsystem1/1(Out1) -> 9-Parameter Regression/1, 3-Parameter Regression/1, 6-Parameter Regression/1
  q/1 -> Subsystem1/1(q)
  qdot/1 -> Subsystem1/2(qdot)
  q_d/1 -> Subsystem1/3(q_d)
  qdot_d/1 -> Subsystem1/4(qdot_d)
  qdotdot_d/1 -> Subsystem1/5(qdotdot_d)
  Integrator/1 -> Manual Switch/1
  Manual Switch/1 -> Matrix Multiply2/2
  Matrix Multiply2/1 -> uFF1/1
  Matrix Multiply1/1 -> Matrix Multiply4/1, Scope3/1, Matrix Multiply3/1
  [du] -> Scope2/1, Matrix Multiply3/2
  Matrix Multiply3/1 -> Scope1/1, Integrator/1
  Matrix Multiply4/1 -> Manual Switch/2
  [u_tot] -> Matrix Multiply4/2

== system Latest_Greatest_vSandberg/Subsystem2/Subsystem/Gravity Gradient/Select ci3 ==
  U : Inport
  C11 : Fcn  Expr=u[3]
  C12 : Fcn  Expr=u[6]
  C13 : Fcn  Expr=u[9]
  Mux2 : Mux  Inputs=3
  U(E) : Outport
  wires:
  C11/1 -> Mux2/1
  C12/1 -> Mux2/2
  C13/1 -> Mux2/3
  U/1 -> C12/1, C11/1, C13/1
  Mux2/1 -> U(E)/1

== system Latest_Greatest_vSandberg/Subsystem2/Subsystem/TAero & Tsolar/Select ci1 ==
  U : Inport
  C11 : Fcn  Expr=u[1]
  C21 : Fcn  Expr=u[4]
  C31 : Fcn  Expr=u[7]
  Mux2 : Mux  Inputs=3
  U(E) : Outport
  wires:
  C11/1 -> Mux2/1
  C21/1 -> Mux2/2
  C31/1 -> Mux2/3
  U/1 -> C21/1, C11/1, C31/1
  Mux2/1 -> U(E)/1

== system Latest_Greatest_vSandberg/Subsystem2/Subsystem/TAero & Tsolar/Sun & Eclipse ==
  note: Sun & Eclipse
  nu : Inport
  DCM : Inport  Port=2
  Atmospheric Force in Body Coords : Product  SaturateOnIntegerOverflow=on  OutDataTypeStr=Inherit: Same as first input
  Eclipse : Fcn  Expr=-cos(u[1])
  Mux : Mux  Inputs=3
  Mux1 : Mux
  Mux2 : Mux  Inputs=3
  Relay : Relay  OnSwitchValue=cos(rho)/cos(betasun)  OffSwitchValue=cos(rho)/cos(betasun)-0.001  OnOutputValue=0  OffOutputValue=1
  Sx (body coordinates) : Fcn  Expr=u[1]*u[10]+u[2]*u[11]+u[3]*u[12]
  Sx (orbit  coordinates) : Fcn  Expr=cos(u[2])*sin(u[1])
  Sy (body coordinates) : Fcn  Expr=u[4]*u[10]+u[5]*u[11]+u[6]*u[12]
  Sy (orbit  coordinates) : Fcn  Expr=sin(u[2])
  Sz (body  coordinates) : Fcn  Expr=u[7]*u[10]+u[8]*u[11]+u[9]*u[12]
  Sz (orbit coordinates) : Fcn  Expr=cos(u[2])*cos(u[1])
  "earth's angular radius, rho" : Constant  Value=rho
  sun beta angle : Constant  Value=betasun
  Sb : Outport
  nu. : Outport  Port=2
  wires:
  Relay/1 -> Atmospheric Force in Body Coords/2
  Eclipse/1 -> Relay/1
  Mux/1 -> Eclipse/1, Sz (orbit coordinates)/1, Sx (orbit  coordinates)/1, Sy (orbit  coordinates)/1
  "earth's angular radius, rho"/1 -> Mux/3
  sun beta angle/1 -> Mux/2
  nu/1 -> Mux/1, nu./1
  Atmospheric Force in Body Coords/1 -> Sb/1
  Mux1/1 -> Sx (body coordinates)/1, Sz (body  coordinates)/1, Sy (body coordinates)/1
  Sx (body coordinates)/1 -> Mux2/1
  Sy (body coordinates)/1 -> Mux2/2
  Sz (body  coordinates)/1 -> Mux2/3
  Mux2/1 -> Atmospheric Force in Body Coords/1
  Sx (orbit  coordinates)/1 -> Mux1/2
  Sy (orbit  coordinates)/1 -> Mux1/3
  Sz (orbit coordinates)/1 -> Mux1/4
  DCM/1 -> Mux1/1

== system Latest_Greatest_vSandberg/Subsystem2/Subsystem1/Gravity Gradient1/Select ci3 ==
  U : Inport
  C11 : Fcn  Expr=u[3]
  C12 : Fcn  Expr=u[6]
  C13 : Fcn  Expr=u[9]
  Mux2 : Mux  Inputs=3
  U(E) : Outport
  wires:
  C11/1 -> Mux2/1
  C12/1 -> Mux2/2
  C13/1 -> Mux2/3
  U/1 -> C12/1, C11/1, C13/1
  Mux2/1 -> U(E)/1

== system Latest_Greatest_vSandberg/Subsystem2/Subsystem1/TAero & Tsolar/Select ci1 ==
  U : Inport
  C11 : Fcn  Expr=u[1]
  C21 : Fcn  Expr=u[4]
  C31 : Fcn  Expr=u[7]
  Mux2 : Mux  Inputs=3
  U(E) : Outport
  wires:
  Mux2/1 -> U(E)/1
  U/1 -> C31/1, C11/1, C21/1
  C31/1 -> Mux2/3
  C21/1 -> Mux2/2
  C11/1 -> Mux2/1

== system Latest_Greatest_vSandberg/Subsystem2/Subsystem1/TAero & Tsolar/Sun & Eclipse ==
  note: Sun & Eclipse
  nu : Inport
  DCM : Inport  Port=2
  Atmospheric Force in Body Coords : Product  SaturateOnIntegerOverflow=on  OutDataTypeStr=Inherit: Same as first input
  Eclipse : Fcn  Expr=-cos(u[1])
  Mux : Mux  Inputs=3
  Mux1 : Mux
  Mux2 : Mux  Inputs=3
  Relay : Relay  OnSwitchValue=cos(rho)/cos(betasun)  OffSwitchValue=cos(rho)/cos(betasun)-0.001  OnOutputValue=0  OffOutputValue=1
  Sx (body coordinates) : Fcn  Expr=u[1]*u[10]+u[2]*u[11]+u[3]*u[12]
  Sx (orbit  coordinates) : Fcn  Expr=cos(u[2])*sin(u[1])
  Sy (body coordinates) : Fcn  Expr=u[4]*u[10]+u[5]*u[11]+u[6]*u[12]
  Sy (orbit  coordinates) : Fcn  Expr=sin(u[2])
  Sz (body  coordinates) : Fcn  Expr=u[7]*u[10]+u[8]*u[11]+u[9]*u[12]
  Sz (orbit coordinates) : Fcn  Expr=cos(u[2])*cos(u[1])
  "earth's angular radius, rho" : Constant  Value=rho
  sun beta angle : Constant  Value=betasun
  Sb : Outport
  nu. : Outport  Port=2
  wires:
  DCM/1 -> Mux1/1
  Sz (orbit coordinates)/1 -> Mux1/4
  Sy (orbit  coordinates)/1 -> Mux1/3
  Sx (orbit  coordinates)/1 -> Mux1/2
  Mux2/1 -> Atmospheric Force in Body Coords/1
  Sz (body  coordinates)/1 -> Mux2/3
  Sy (body coordinates)/1 -> Mux2/2
  Sx (body coordinates)/1 -> Mux2/1
  Mux1/1 -> Sy (body coordinates)/1, Sz (body  coordinates)/1, Sx (body coordinates)/1
  Atmospheric Force in Body Coords/1 -> Sb/1
  nu/1 -> nu./1, Mux/1
  sun beta angle/1 -> Mux/2
  "earth's angular radius, rho"/1 -> Mux/3
  Mux/1 -> Sy (orbit  coordinates)/1, Sx (orbit  coordinates)/1, Sz (orbit coordinates)/1, Eclipse/1
  Eclipse/1 -> Relay/1
  Relay/1 -> Atmospheric Force in Body Coords/2

== system Latest_Greatest_vSandberg/Subsystem5/OBSERVERS (MASK THIS SUBSYSTEM AS CLASS DEMO)1/Subsystem/Subsystem ==
  Luenberger : Inport
  PID : Inport  Port=2
  Estimated Euler Angles (deg) : Scope
      settings: StopFcn=|
      | %Simulink figure properties
      | shh=get(0,'ShowHiddenHandles');
      | set(0,'ShowHiddenHandles','On')
      | set(gcf,'menubar','figure')
      | set(gcf,'CloseRequestFcn','closereq')
      | set(gcf,'DefaultLineClipping','Off')
      | set(0,'ShowHiddenHandles',shh)
  Reshape : Reshape
  Reshape2 : Reshape  OutputDimensions=[1,9]
  Reshape3 : Reshape  OutputDimensions=[1,9]
  Sum2 : Sum  Inputs=|+-
  Sum3 : Sum  Inputs=|+-
  To Workspace : ToWorkspace  VariableName=EstimatedEuler  SampleTime=-1
  To Workspace1 : ToWorkspace  VariableName=EstimationError  SampleTime=-1
  To Workspace2 : ToWorkspace  VariableName=PIDoEstimationError  SampleTime=-1
  degrees-to-radians1 : Gain  Gain=180/pi
  degrees-to-radians2 : Gain  Gain=180/pi
  wires:
  degrees-to-radians2/1 -> Reshape/1
  Reshape/1 -> Estimated Euler Angles (deg)/1, Sum3/2
  PID/1 -> degrees-to-radians2/1
  Sum3/1 -> To Workspace2/1
  Luenberger/1 -> degrees-to-radians1/1
  Reshape3/1 -> To Workspace1/1
  Reshape2/1 -> To Workspace/1
  [ActualEuler] -> Sum3/1, Sum2/1
  Sum2/1 -> Reshape3/1
  degrees-to-radians1/1 -> Reshape2/1, Sum2/2

== system Latest_Greatest_vSandberg/Subsystem5/OBSERVERS (MASK THIS SUBSYSTEM AS CLASS DEMO)1/Subsystem/Subsystem1 ==
  In1 : Inport
  Gain : Gain  Gain=Iinv  Multiplication=Matrix(K*u)
  Out1 : Outport  VectorParamsAs1DForOutWhenUnconnected=off
  wires:
  In1/1 -> Gain/1
  Gain/1 -> Out1/1

== system Latest_Greatest_vSandberg/Subsystem5/OBSERVERS (MASK THIS SUBSYSTEM AS CLASS DEMO)1/Subsystem/Subsystem10 ==
  In1 : Inport
  Gain : Gain  Gain=Kdo
  Out1 : Outport  VectorParamsAs1DForOutWhenUnconnected=off
  wires:
  Gain/1 -> Out1/1
  In1/1 -> Gain/1

== system Latest_Greatest_vSandberg/Subsystem5/OBSERVERS (MASK THIS SUBSYSTEM AS CLASS DEMO)1/Subsystem/Subsystem11 ==
  In1 : Inport
  Gain : Gain  Gain=Kpo
  Out1 : Outport  VectorParamsAs1DForOutWhenUnconnected=off
  wires:
  In1/1 -> Gain/1
  Gain/1 -> Out1/1

== system Latest_Greatest_vSandberg/Subsystem5/OBSERVERS (MASK THIS SUBSYSTEM AS CLASS DEMO)1/Subsystem/Subsystem2 ==
  In1 : Inport
  Gain : Gain  Gain=Kdo
  Out1 : Outport  VectorParamsAs1DForOutWhenUnconnected=off
  wires:
  Gain/1 -> Out1/1
  In1/1 -> Gain/1

== system Latest_Greatest_vSandberg/Subsystem5/OBSERVERS (MASK THIS SUBSYSTEM AS CLASS DEMO)1/Subsystem/Subsystem5 ==
  In1 : Inport
  Gain : Gain  Gain=Kio
  Out1 : Outport  VectorParamsAs1DForOutWhenUnconnected=off
  wires:
  Gain/1 -> Out1/1
  In1/1 -> Gain/1

== system Latest_Greatest_vSandberg/Subsystem5/OBSERVERS (MASK THIS SUBSYSTEM AS CLASS DEMO)1/Subsystem/Subsystem6 ==
  In1 : Inport
  Gain : Gain  Gain=Iinv  Multiplication=Matrix(K*u)
  Out1 : Outport  VectorParamsAs1DForOutWhenUnconnected=off
  wires:
  Gain/1 -> Out1/1
  In1/1 -> Gain/1

== system Latest_Greatest_vSandberg/Subsystem5/OBSERVERS (MASK THIS SUBSYSTEM AS CLASS DEMO)1/Subsystem/Subsystem7 ==
  In1 : Inport
  Gain : Gain  Gain=Iinv  Multiplication=Matrix(K*u)
  Out1 : Outport  VectorParamsAs1DForOutWhenUnconnected=off
  wires:
  In1/1 -> Gain/1
  Gain/1 -> Out1/1

== system Latest_Greatest_vSandberg/Subsystem5/OBSERVERS (MASK THIS SUBSYSTEM AS CLASS DEMO)1/Subsystem/Subsystem8 ==
  In1 : Inport
  Gain : Gain  Gain=Kio
  Out1 : Outport  VectorParamsAs1DForOutWhenUnconnected=off
  wires:
  Gain/1 -> Out1/1
  In1/1 -> Gain/1

== system Latest_Greatest_vSandberg/Subsystem5/OBSERVERS (MASK THIS SUBSYSTEM AS CLASS DEMO)1/Subsystem/Subsystem9 ==
  In1 : Inport
  Gain : Gain  Gain=Kpo
  Out1 : Outport  VectorParamsAs1DForOutWhenUnconnected=off
  wires:
  In1/1 -> Gain/1
  Gain/1 -> Out1/1

== system Latest_Greatest_vSandberg/CMGs/Subsystem3/Subsystem4/Subsystem3/Subsystem ==
  T : Inport
  " LU Inverse" : dspinverses/ LU Inverse  mask(LU Inverse){}
      mask Display:
      | % This is a new mask on top of the base mask.
      | % Use "View base mask" link below to see the base mask.
      | disp('LU Inverse')
  Interpreted MATLAB Function : MATLABFcn  Commented=on  MATLABFcn=u^-1
      mask Display: disp('[T]^-1')
  Interpreted MATLAB Function1 : MATLABFcn  MATLABFcn=1.\u
      mask Display: disp('1\T')
  Interpreted MATLAB Function2 : MATLABFcn  MATLABFcn=inv(u)
      mask Display: disp('inv([T])')
  Interpreted MATLAB Function3 : MATLABFcn  MATLABFcn=pinv(u)
      mask Display: disp('pinv([T])')
  Interpreted MATLAB Function4 : MATLABFcn  MATLABFcn=det(u)
      mask Display: disp('det([T])')
  Manual Switch : ManualSwitch  CurrentSetting=0
  Manual Switch1 : ManualSwitch
  Manual Switch2 : ManualSwitch
  Manual Switch3 : ManualSwitch
  Reshape : Reshape  OutputDimensionality=Customize  OutputDimensions=[9,9]
  Reshape1 : Reshape  OutputDimensionality=Customize  OutputDimensions=[9,9]
  inv(T) : Outport
  det(T) : Outport  Port=2
  wires:
  Interpreted MATLAB Function/1 -> Manual Switch/1
  Interpreted MATLAB Function1/1 -> Manual Switch/2
  Manual Switch/1 -> Manual Switch1/1
  Interpreted MATLAB Function2/1 -> Manual Switch1/2
  Manual Switch1/1 -> Manual Switch2/1
  Interpreted MATLAB Function3/1 -> Manual Switch2/2
  Manual Switch2/1 -> Reshape1/1
  T/1 -> Reshape/1
  Reshape/1 -> Interpreted MATLAB Function/1, Interpreted MATLAB Function1/1, Interpreted MATLAB Function4/1, " LU Inverse"/1, Interpreted MATLAB Function3/1, Interpreted MATLAB Function2/1
  " LU Inverse"/1 -> Manual Switch3/2
  Manual Switch3/1 -> inv(T)/1
  Interpreted MATLAB Function4/1 -> det(T)/1
  Reshape1/1 -> Manual Switch3/1
